simulink model "dynamics_scheme"  (R2021b)
settings: Solver=VariableStepAuto  StartTime=0.0  StopTime=10.0  RelTol=1e-3
undefined symbols (not defined in the file): angles, F_force, velocity
settings Model: Creator=szymon_kubuntu  LastModifiedBy=szymon_kubuntu

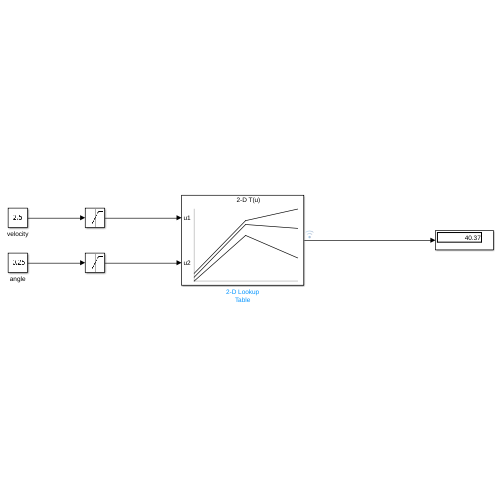
[thumbnail: Simulink's stored preview of the top-level diagram]
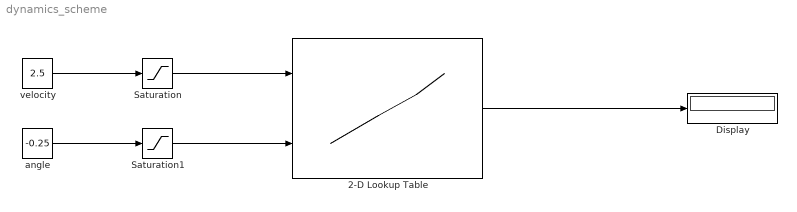
== system dynamics_scheme ==
  2-D Lookup Table : Lookup_n-D  BreakpointsForDimension1=velocity  BreakpointsForDimension2=angles  Table=F_force  InternalRulePriority=Speed  RndMeth=Simplest  InputSameDT=on
      settings: InputPortMap=u0,u1
  Display : Display
  Saturation : Saturate  UpperLimit=832/3.6  LowerLimit=0
  Saturation1 : Saturate  UpperLimit=deg2rad(15)  LowerLimit=deg2rad(-15)
  angle : Constant  Value=-0.25
  velocity : Constant  Value=2.5
  wires:
  angle/1 -> Saturation1/1
  velocity/1 -> Saturation/1
  2-D Lookup Table/1 -> Display/1
  Saturation/1 -> 2-D Lookup Table/1
  Saturation1/1 -> 2-D Lookup Table/2
